simulink model "TestPieroHW"  (R2024b)
settings: Solver=VariableStepAuto  StartTime=0.0  StopTime=10.0  RelTol=1e-3
settings Model: Creator=Chenfu  LastModifiedBy=Chenfu

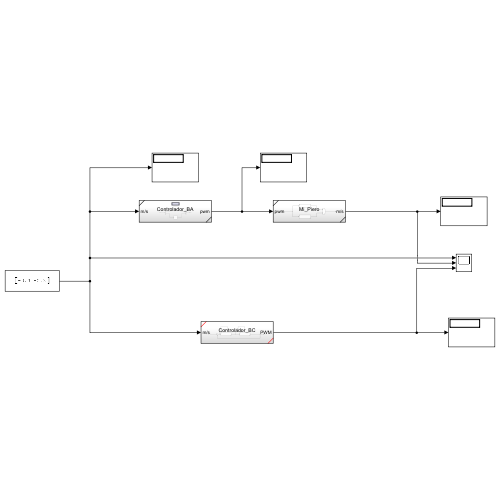
[thumbnail: Simulink's stored preview of the top-level diagram]
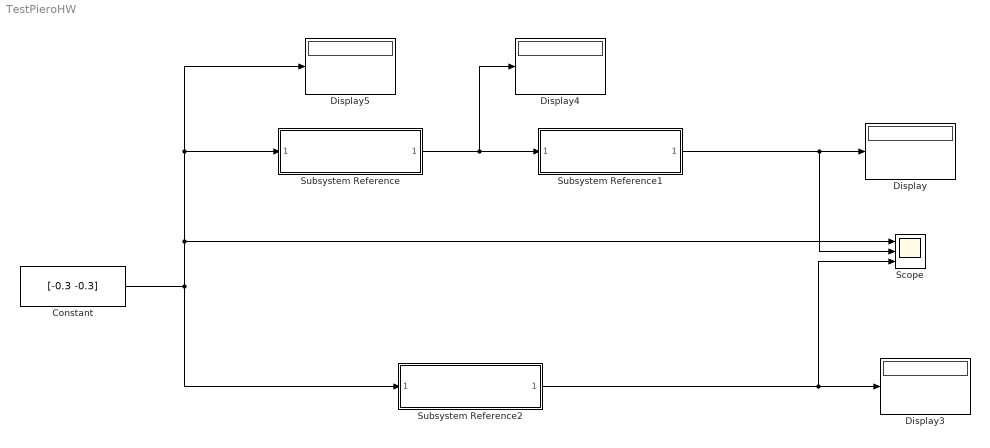
== system TestPieroHW ==
  Constant : Constant  Value=[-0.3 -0.3]
  Display{,3..5} (4 alike) : Display
  Scope : Scope  NumInputPorts=3
  Subsystem Reference : Subsystem  ReferencedSubsystem=Controlador_BA
  Subsystem Reference1 : Subsystem  ReferencedSubsystem=Mi_Piero
  Subsystem Reference2 : Subsystem  ReferencedSubsystem=Controlador_BC
  wires:
  Subsystem Reference/1 -> Display4/1, Subsystem Reference1/1
  Subsystem Reference1/1 -> Scope/2, Display/1
  Constant/1 -> Subsystem Reference2/1, Subsystem Reference/1, Display5/1, Scope/1
  Subsystem Reference2/1 -> Scope/3, Display3/1
